simulink model "pmsm_model_Lab3_MTPA_st_R2020a"  (R2023a)
settings: Solver=ode45  StartTime=0.0  StopTime=Tf  FixedStep=Tsim  MaxStep=Tsim  MinStep=Tsim/100  RelTol=1e-3
values from neighbouring files (symbols this model uses):
  C32 = [ 1       0 ... (first row only)    [pmsm_param_Lab1_2025.m]    (also in pmsm_param_Lab2_2025_st.m; pmsm_param_Lab3_st.m; pmsm_param_Lab4_2024_st.m)
  C32inv = 2/3*[1    -1/2        -1/2 ... (first row only)    [pmsm_param_Lab1_2025.m]    (also in pmsm_param_Lab2_2025_st.m; pmsm_param_Lab3_st.m; pmsm_param_Lab4_2024_st.m)
  C33 = C32*C32inv    [pmsm_param_Lab1_2025.m]    (also in pmsm_param_Lab2_2025_st.m; pmsm_param_Lab3_st.m; pmsm_param_Lab4_2024_st.m)
  Cb = 500e-6    (= 0.0005)    [pmsm_param_Lab3_st.m]    (also in pmsm_param_Lab4_2024_st.m)
  dTm0 = 0.20*Tmrated    (= 48)    [pmsm_param_Lab2_2025_st.m]    (also in pmsm_param_Lab3_st.m; pmsm_param_Lab4_2024_st.m = 120)
  Dyno = 1    [pmsm_param_Lab3_st.m]    (also in pmsm_param_Lab4_2024_st.m = 0)
  f = 15e-3    (= 0.015)    [pmsm_param_Lab1_2025.m]    (also in pmsm_param_Lab2_2025_st.m; pmsm_param_Lab3_st.m; pmsm_param_Lab4_2024_st.m)
  GVSI = 1    [pmsm_param_Lab2_2025_st.m]    (also in pmsm_param_Lab3_st.m; pmsm_param_Lab4_2024_st.m)
  Id0 = 0    [pmsm_param_Lab1_2025.m]    (also in pmsm_param_Lab2_2025_st.m; pmsm_param_Lab3_st.m = interp1(Tref,Idopt,Tm0); pmsm_param_Lab4_2024_st.m = interp1(Tref,Idopt,Tm0))
  Idc0 = Pe0/VDC    [pmsm_param_Lab3_st.m]    (also in pmsm_param_Lab4_2024_st.m)
  Idopt = zeros(1,NT)    [pmsm_param_Lab3_st.m]    (also in pmsm_param_Lab4_2024_st.m)
  Iq0 = 2/3*Tm0/(Pp*Psif)    (= 0)    [pmsm_param_Lab1_2025.m]    (also in pmsm_param_Lab2_2025_st.m = 119.926066866; pmsm_param_Lab3_st.m = interp1(Tref,Iqopt,Tm0); pmsm_param_Lab4_2024_st.m = interp1(Tref,Iqopt,Tm0))
  Iqopt = zeros(1,NT)    [pmsm_param_Lab3_st.m]    (also in pmsm_param_Lab4_2024_st.m)
  J = 100e-3    (= 0.1)    [pmsm_param_Lab1_2025.m]    (also in pmsm_param_Lab2_2025_st.m; pmsm_param_Lab3_st.m; pmsm_param_Lab4_2024_st.m)
  Kid = Kpd / tid    (= 282.743237724)    [pmsm_param_Lab2_2025_st.m]    (also in pmsm_param_Lab3_st.m = 180; pmsm_param_Lab4_2024_st.m = 180)
  Kiq = Kpq / tiq    (= 282.743237724)    [pmsm_param_Lab2_2025_st.m]    (also in pmsm_param_Lab3_st.m = 180; pmsm_param_Lab4_2024_st.m = 180)
  kL = 0.750    (= 0.75)    [pmsm_param_Lab1_2025.m]    (also in pmsm_param_Lab2_2025_st.m; pmsm_param_Lab3_st.m; pmsm_param_Lab4_2024_st.m)
  Kpd = (3*Ld0) / tr    (= 6.28318306054)    [pmsm_param_Lab2_2025_st.m]    (also in pmsm_param_Lab3_st.m = 3; pmsm_param_Lab4_2024_st.m = 3)
  Kpq = (3 * Lq0) / tr    (= 3.14159153027)    [pmsm_param_Lab2_2025_st.m]    (also in pmsm_param_Lab3_st.m = 6; pmsm_param_Lab4_2024_st.m = 6)
  Lb = 20e-6    (= 2e-05)    [pmsm_param_Lab3_st.m]    (also in pmsm_param_Lab4_2024_st.m)
  Ld0 = 2.0*Ld    (= 0.002)    [pmsm_param_Lab2_2025_st.m]    (also in pmsm_param_Lab3_st.m = 0.001; pmsm_param_Lab4_2024_st.m = 0.001)
  Lq0 = 0.5*Lq    (= 0.001)    [pmsm_param_Lab2_2025_st.m]    (also in pmsm_param_Lab3_st.m = 0.002; pmsm_param_Lab4_2024_st.m = 0.002)
  Pe0 = 3/2*(Vd0*Id0+Vq0*Iq0)    [pmsm_param_Lab2_2025_st.m]    (also in pmsm_param_Lab3_st.m; pmsm_param_Lab4_2024_st.m)
  Pp = 4    [pmsm_param_Lab1_2025.m]    (also in pmsm_param_Lab2_2025_st.m; pmsm_param_Lab3_st.m; pmsm_param_Lab4_2024_st.m)
  Psid0 = interpn(Idv,Iqv,Psidd,Id0,Iq0)    [pmsm_param_Lab1_2025.m]    (also in pmsm_param_Lab2_2025_st.m; pmsm_param_Lab3_st.m; pmsm_param_Lab4_2024_st.m)
  Psif0 = 1.0*Psif    (= 0.167)    [pmsm_param_Lab2_2025_st.m]    (also in pmsm_param_Lab3_st.m; pmsm_param_Lab4_2024_st.m)
  Psiq0 = interpn(Idv,Iqv,Psiqq,Id0,Iq0)    [pmsm_param_Lab1_2025.m]    (also in pmsm_param_Lab2_2025_st.m; pmsm_param_Lab3_st.m; pmsm_param_Lab4_2024_st.m)
  Qbat = 72*3600    (= 259200)    [pmsm_param_Lab3_st.m]    (also in pmsm_param_Lab4_2024_st.m)
  RateTm = 10000    [pmsm_param_Lab3_st.m]    (also in pmsm_param_Lab4_2024_st.m)
  rb = 80e-3    (= 0.08)    [pmsm_param_Lab3_st.m]    (also in pmsm_param_Lab4_2024_st.m)
  Rs = 60e-3    (= 0.06)    [pmsm_param_Lab1_2025.m]    (also in pmsm_param_Lab2_2025_st.m; pmsm_param_Lab3_st.m; pmsm_param_Lab4_2024_st.m)
  Rs0 = 1.5*Rs    (= 0.09)    [pmsm_param_Lab2_2025_st.m]    (also in pmsm_param_Lab3_st.m = 0.06; pmsm_param_Lab4_2024_st.m = 0.06)
  SOC0 = 0.50    (= 0.5)    [pmsm_param_Lab3_st.m]    (also in pmsm_param_Lab4_2024_st.m)
  Thetae0 = 0    [pmsm_param_Lab1_2025.m]    (also in pmsm_param_Lab2_2025_st.m; pmsm_param_Lab3_st.m; pmsm_param_Lab4_2024_st.m)
  Tm0 = (kL+f)*Wm0    (= 0)    [pmsm_param_Lab1_2025.m]    (also in pmsm_param_Lab2_2025_st.m = 120.165919; pmsm_param_Lab3_st.m = 192.2654704; pmsm_param_Lab4_2024_st.m)
  Tp = 100e-6    (= 0.0001)    [pmsm_param_Lab2_2025_st.m]    (also in pmsm_param_Lab3_st.m; pmsm_param_Lab4_2024_st.m)
  Tref = -Tmax:Tmax/100:Tmax    [pmsm_param_Lab3_st.m]    (also in pmsm_param_Lab4_2024_st.m)
  Ts = Tsim    [pmsm_param_Lab2_2025_st.m]    (also in pmsm_param_Lab3_st.m = 0.0001; pmsm_param_Lab4_2024_st.m = 0.0001)
  Tsim = 1e-6    (= 1e-06)    [pmsm_param_Lab1_2025.m]    (also in pmsm_param_Lab2_2025_st.m = min([Tp Ts])/100; pmsm_param_Lab3_st.m = min([Tp Ts])/100; pmsm_param_Lab4_2024_st.m = min([Tp Ts])/100)
  TSS = Tstep+0.050    (= 0.1)    [pmsm_param_Lab3_st.m]    (also in pmsm_param_Lab4_2024_st.m)
  Tstep = 0.10    (= 0.1)    [pmsm_param_Lab2_2025_st.m]    (also in pmsm_param_Lab3_st.m = 0.05; pmsm_param_Lab4_2024_st.m = 0.05)
  Ud0 = Rs*Id0    (= 0)    [pmsm_param_Lab2_2025_st.m]    (also in pmsm_param_Lab3_st.m; pmsm_param_Lab4_2024_st.m)
  Uq0 = Rs*Iq0    (= 7.19556401196)    [pmsm_param_Lab2_2025_st.m]    (also in pmsm_param_Lab3_st.m = 11.5129024191; pmsm_param_Lab4_2024_st.m = Rs*Iq0)
  Vd0 = Rs*Id0-Pp*Psiq0*Wm0    [pmsm_param_Lab1_2025.m]    (also in pmsm_param_Lab2_2025_st.m = Ud0-Pp*Psiq0*Wm0; pmsm_param_Lab3_st.m = Ud0-Pp*Psiq0*Wm0; pmsm_param_Lab4_2024_st.m = Ud0-Pp*Psiq0*Wm0)
  VDC = 800    [pmsm_param_Lab2_2025_st.m]    (also in pmsm_param_Lab3_st.m; pmsm_param_Lab4_2024_st.m)
  VDC0 = 0.8*VDC    (= 640)    [pmsm_param_Lab3_st.m]    (also in pmsm_param_Lab4_2024_st.m)
  Vp = VDC/2    (= 400)    [pmsm_param_Lab2_2025_st.m]    (also in pmsm_param_Lab3_st.m; pmsm_param_Lab4_2024_st.m)
  Vq0 = Rs*Iq0+Pp*Psid0*Wm0    [pmsm_param_Lab1_2025.m]    (also in pmsm_param_Lab2_2025_st.m = Uq0+Pp*Psid0*Wm0; pmsm_param_Lab3_st.m = Uq0+Pp*Psid0*Wm0; pmsm_param_Lab4_2024_st.m = Uq0+Pp*Psid0*Wm0)
  Wm0 = 0    [pmsm_param_Lab1_2025.m]    (also in pmsm_param_Lab2_2025_st.m = 157.079632679; pmsm_param_Lab3_st.m = 251.327412287; pmsm_param_Lab4_2024_st.m)
undefined symbols (not defined in the file or in its folder): Idd, Idrop, Iqq, Isw, Psidv, Psiqv, SwLoss, Vdrop
libraries: simulink x11, spsTHDLib x1
(part 2 of 2)

== system pmsm_model_Lab3_MTPA_st_R2020a/VSI/VSI_Power/Subsystem1/Subsystem2/Subsystem1 ==
  U : Inport
  Compare To Constant : simulink/Logic and Bit Operations/Compare To Constant  relop=>  const=VDC0  OutDataTypeStr=uint8
  Memory : Memory
  Sum : Sum  Inputs=+-|
  Out1 : Outport
  wires:
  U/1 -> Memory/1, Sum/1
  Sum/1 -> Compare To Constant/1
  Memory/1 -> Sum/2
  Compare To Constant/1 -> Out1/1

== system pmsm_model_Lab3_MTPA_st_R2020a/VSI/VSI_Power/Subsystem1/Subsystem3/Subsystem ==
  U : Inport
  Compare To Constant : simulink/Logic and Bit Operations/Compare To Constant  relop=<  const=-VDC0  OutDataTypeStr=uint8
  Memory : Memory
  Sum : Sum  Inputs=+-|
  Out1 : Outport
  wires:
  Memory/1 -> Sum/2
  Sum/1 -> Compare To Constant/1
  U/1 -> Memory/1, Sum/1
  Compare To Constant/1 -> Out1/1

== system pmsm_model_Lab3_MTPA_st_R2020a/VSI/VSI_Power/Subsystem1/Subsystem3/Subsystem1 ==
  U : Inport
  Compare To Constant : simulink/Logic and Bit Operations/Compare To Constant  relop=>  const=VDC0  OutDataTypeStr=uint8
  Memory : Memory
  Sum : Sum  Inputs=+-|
  Out1 : Outport
  wires:
  U/1 -> Memory/1, Sum/1
  Sum/1 -> Compare To Constant/1
  Memory/1 -> Sum/2
  Compare To Constant/1 -> Out1/1

== matlab function pmsm_model_Lab3_MTPA_st_R2020a/PMSM/dq-PMSM ==
  data: vd input; dPsid output; vq input; id input; iq input; Psid input; Psiq input; Omega input; TL input; dPsiq output; dOmega output; dTheta output; Rs input; Pp parameter; f parameter; J parameter; Tm output
function [dPsid, dPsiq, dOmega, dTheta, Tm] = PMSM(vd, vq, id, iq, Psid, Psiq, Omega, TL, Rs, Pp, f, J)

w=Pp*Omega;
Tm=(3/2)*Pp*(Psid*iq-Psiq*id);   % Clarke
% Tm=p*(Psid*iq-Psiq*id);       % Concordia

dPsid=vd-Rs*id+w*Psiq;
dPsiq=vq-Rs*iq-w*Psid;
dOmega=(Tm-f*Omega-TL)/J;
dTheta=w;

== matlab function pmsm_model_Lab3_MTPA_st_R2020a/Control/Ctrl ==
  data: method input; idref input; idm input; iqref input; iqm input; we input; VDC input; Pp parameter; Psif0 parameter; Ld0 parameter; Lq0 parameter; Rs0 parameter; Ts parameter; vd output; vq output; Kpd parameter; Kpq parameter; Kid parameter; Kiq parameter; Id0 parameter; Iq0 parameter; Ud0 parameter; Uq0 parameter; Tm0 parameter; Vd0 parameter; Vq0 parameter; load output
function [vd, vq, load]  = Ctrl(method, idref, idm, iqref, iqm, we, VDC, Pp, Psif0, Ld0, Lq0, Rs0, Ts, Kpd, Kpq, Kid, Kiq, Id0, Iq0, Ud0, Uq0, Tm0, Vd0, Vq0)

persistent interrd interrq exetime

method=fix(method);
if method<0, method=0; end
if method>9, method=9; end

if isempty(interrd), if method==0, interrd = Vd0; else interrd = Ud0; end, end
if isempty(interrq), if method==0, interrq = Vq0; else interrq = Uq0; end, end
if isempty(exetime), exetime = 0; end

tic

switch method
    case 0   % PI
        errd=idref-idm;
        errq=iqref-iqm;
        interrd=interrd+Kid*errd*Ts;
        interrq=interrq+Kiq*errq*Ts;
        vd=Kpd*errd+interrd;
        vq=Kpq*errq+interrq;
    case 1   % PI+feedback decoupling
        errd=idref-idm;
        errq=iqref-iqm;
        interrd=interrd+Kid*errd*Ts;
        interrq=interrq+Kiq*errq*Ts;
        vd=Kpd*errd+interrd-Lq0*iqm*we;
        vq=Kpq*errq+interrq+(Psif0+Ld0*idm)*we;
    case 2   % Deadbeat MPC
        vd=Rs0*idm - we*Lq0*iqm + Ld0/Ts*(idref - idm) + Kpd*(idref - idm);
        vq=Rs0*iqm + we*(Ld0*idm + Psif0) + Lq0/Ts*(iqref - iqm) + Kpq*(iqref - iqm);
        V_tot = sqrt(vd^2 + vq^2); %We use THIPWM here, U can not pass the limit
        Vmax = VDC / sqrt(3);
        if (V_tot > Vmax)
            vd = vd*Vmax/V_tot;
            vq = vq*Vmax/V_tot;
        end
    case 3   % CCS-MPC + decoupling + gradient?
        vd=0;
        vq=0;       
    otherwise
        vd=0;
        vq=0;
end

exetime=exetime+toc;
load=exetime;
